simulink model "Roadsense_TrajectoryController"  (R2025b)
settings: Solver=FixedStepDiscrete  StartTime=0.0  StopTime=1.0  FixedStep=RsTsBase  RelTol=1e-3
undefined symbols (not defined in the file or in its folder): RsMaxPlanPoints, RsTsControl
settings Model: DataDictionary=Roadsense_Data.sldd  Creator=ragur  LastModifiedBy=ragur

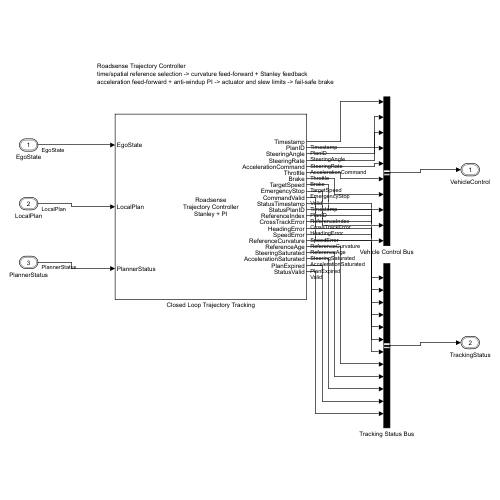
[thumbnail: Simulink's stored preview of the top-level diagram]
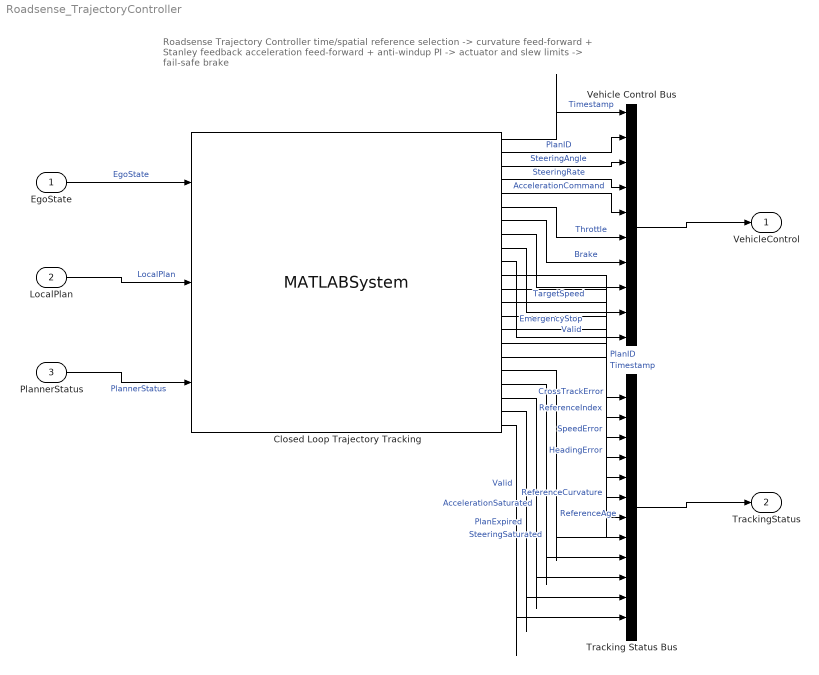
== system Roadsense_TrajectoryController ==
  note: Roadsense Trajectory Controller
      | time/spatial reference selection -> curvature feed-forward + Stanley feedback
      | acceleration feed-forward + anti-windup PI -> actuator and slew limits -> fail-safe brake
  EgoState : Inport  OutDataTypeStr=Bus: RsEgoStateBus  PortDimensions=1  SampleTime=RsTsControl
  LocalPlan : Inport  Port=2  OutDataTypeStr=Bus: RsLocalPlanBus  PortDimensions=1  SampleTime=RsTsControl
  PlannerStatus : Inport  Port=3  OutDataTypeStr=Bus: RsPlannerStatusBus  PortDimensions=1  SampleTime=RsTsControl
  Closed Loop Trajectory Tracking : MATLABSystem  System=RoadsenseTrajectoryControllerSystem  MaxPlanPoints=double(RsMaxPlanPoints)  SampleTime=RsTsControl  Wheelbase=RsControllerWheelbase  LateralGain=RsControllerLateralGain  HeadingGain=RsControllerHeadingGain  SofteningSpeed=RsControllerSofteningSpeed  SpeedKp=RsControllerSpeedKp  SpeedKi=RsControllerSpeedKi  IntegralLimit=RsControllerIntegralLimit  MaximumSteering=RsControllerMaximumSteering  MaximumSteeringRate=RsControllerMaximumSteeringRate  MaximumAcceleration=RsControllerMaximumAcceleration  MaximumDeceleration=RsControllerMaximumDeceleration  AccelerationSlew=RsControllerAccelerationSlew  PreviewTime=RsControllerPreviewTime  PlanGrace=RsControllerPlanGrace  SimulateUsing=Code generation
      mask Type: RoadsenseTrajectoryControllerSystem
  Tracking Status Bus : BusCreator  Inputs=12  OutDataTypeStr=Bus: RsTrackingStatusBus
  Vehicle Control Bus : BusCreator  Inputs=10  OutDataTypeStr=Bus: RsVehicleControlBus
  VehicleControl : Outport  OutDataTypeStr=Bus: RsVehicleControlBus
  TrackingStatus : Outport  Port=2  OutDataTypeStr=Bus: RsTrackingStatusBus
  wires:
  EgoState/1 -> Closed Loop Trajectory Tracking/1  "EgoState"
  LocalPlan/1 -> Closed Loop Trajectory Tracking/2  "LocalPlan"
  PlannerStatus/1 -> Closed Loop Trajectory Tracking/3  "PlannerStatus"
  Closed Loop Trajectory Tracking/1 -> Vehicle Control Bus/1  "Timestamp"
  Closed Loop Trajectory Tracking/2 -> Vehicle Control Bus/2  "PlanID"
  Closed Loop Trajectory Tracking/3 -> Vehicle Control Bus/3  "SteeringAngle"
  Closed Loop Trajectory Tracking/4 -> Vehicle Control Bus/4  "SteeringRate"
  Closed Loop Trajectory Tracking/5 -> Vehicle Control Bus/5  "AccelerationCommand"
  Closed Loop Trajectory Tracking/6 -> Vehicle Control Bus/6  "Throttle"
  Closed Loop Trajectory Tracking/7 -> Vehicle Control Bus/7  "Brake"
  Closed Loop Trajectory Tracking/8 -> Vehicle Control Bus/8  "TargetSpeed"
  Closed Loop Trajectory Tracking/9 -> Vehicle Control Bus/9  "EmergencyStop"
  Closed Loop Trajectory Tracking/10 -> Vehicle Control Bus/10  "Valid"
  Closed Loop Trajectory Tracking/11 -> Tracking Status Bus/1  "Timestamp"
  Closed Loop Trajectory Tracking/12 -> Tracking Status Bus/2  "PlanID"
  Closed Loop Trajectory Tracking/13 -> Tracking Status Bus/3  "ReferenceIndex"
  Closed Loop Trajectory Tracking/14 -> Tracking Status Bus/4  "CrossTrackError"
  Closed Loop Trajectory Tracking/15 -> Tracking Status Bus/5  "HeadingError"
  Closed Loop Trajectory Tracking/16 -> Tracking Status Bus/6  "SpeedError"
  Closed Loop Trajectory Tracking/17 -> Tracking Status Bus/7  "ReferenceCurvature"
  Closed Loop Trajectory Tracking/18 -> Tracking Status Bus/8  "ReferenceAge"
  Closed Loop Trajectory Tracking/19 -> Tracking Status Bus/9  "SteeringSaturated"
  Closed Loop Trajectory Tracking/20 -> Tracking Status Bus/10  "AccelerationSaturated"
  Closed Loop Trajectory Tracking/21 -> Tracking Status Bus/11  "PlanExpired"
  Closed Loop Trajectory Tracking/22 -> Tracking Status Bus/12  "Valid"
  Vehicle Control Bus/1 -> VehicleControl/1
  Tracking Status Bus/1 -> TrackingStatus/1
